simulink model "ASM_Traffic_V2X_Complete_Model_2"  (R2019a)
settings: Solver=ode1  StartTime=SIM.tstart.v  StopTime=Inf  FixedStep=SIM.StepSize.v  RelTol=1e-3
PostLoadFcn:
  | if any(exist('dsrtsu_mdlpostloadfcn', 'file') ~= 0), dsrtsu_mdlpostloadfcn('Execute', bdroot); end
  | try, asm_mdl_postloadfcn(bdroot, 'UpdateModel', 2200); catch, disp(lasterr); end,
undefined symbols (not defined in the file): _SensorPnts_1, _SensorPnts_13, _SensorPnts_17, _SensorPnts_21, _SensorPnts_25, _SensorPnts_29, _SensorPnts_33, _SensorPnts_37, _SensorPnts_41, _SensorPnts_45, _SensorPnts_49, _SensorPnts_5, _SensorPnts_53, _SensorPnts_57, _SensorPnts_9, _to_, CPT, G5A, ITS, MDL, rad, s_to_rpm, SIM
libraries: simulink x169, ASM_VehicleDynamics_lib x126, ASM_Traffic_lib x83, ASM_Utils_lib x49, mdbs x45, ASM_Environment_lib x17, dspindex x12, dsaV2xLibraryAux x10, dsmpblib x6, dsaV2xAsn1Library x4, dsaV2xLibrary x4, ASM_BrakeHydraulics_lib x4
(part 23 of 36)

== system ASM_Traffic_V2X_Complete_Model_2/MDLUserInterface/SoftECU/MDL_DISP/SoftECU_ACC/Dist_Long[m] ==
  In1 : Inport
  Out1 : Outport
  wires:
  In1/1 -> Out1/1

== system ASM_Traffic_V2X_Complete_Model_2/MDLUserInterface/SoftECU/MDL_DISP/SoftECU_ACC/Distance_Set[m] ==
  In1 : Inport
  Out1 : Outport
  wires:
  In1/1 -> Out1/1

== system ASM_Traffic_V2X_Complete_Model_2/MDLUserInterface/SoftECU/MDL_DISP/SoftECU_ACC/FCW[0Off|1On] ==
  In1 : Inport
  Out1 : Outport
  wires:
  In1/1 -> Out1/1

== system ASM_Traffic_V2X_Complete_Model_2/MDLUserInterface/SoftECU/MDL_DISP/SoftECU_ACC/State_ACC[0Off|1On] ==
  In1 : Inport
  Out1 : Outport
  wires:
  In1/1 -> Out1/1

== system ASM_Traffic_V2X_Complete_Model_2/MDLUserInterface/SoftECU/MDL_DISP/SoftECU_ACC/Sw_BrakeMode[1Comfort|2AEBOnly|3AEBOff] ==
  In1 : Inport
  Out1 : Outport
  wires:
  In1/1 -> Out1/1

== system ASM_Traffic_V2X_Complete_Model_2/MDLUserInterface/SoftECU/MDL_DISP/SoftECU_ACC/TTC[s] ==
  In1 : Inport
  Out1 : Outport
  wires:
  In1/1 -> Out1/1

== system ASM_Traffic_V2X_Complete_Model_2/MDLUserInterface/SoftECU/MDL_DISP/SoftECU_ACC/Target_Detected[0|1] ==
  In1 : Inport
  Out1 : Outport
  wires:
  In1/1 -> Out1/1

== system ASM_Traffic_V2X_Complete_Model_2/MDLUserInterface/SoftECU/MDL_DISP/SoftECU_ACC/Trq_Request_Brake_ACC[Nm] ==
  In1 : Inport
  Out1 : Outport
  wires:
  In1/1 -> Out1/1

== system ASM_Traffic_V2X_Complete_Model_2/MDLUserInterface/SoftECU/MDL_DISP/SoftECU_ACC/Trq_Request_Engine_ACC[Nm] ==
  In1 : Inport
  Out1 : Outport
  wires:
  In1/1 -> Out1/1

== system ASM_Traffic_V2X_Complete_Model_2/MDLUserInterface/SoftECU/MDL_DISP/SoftECU_ACC/v_Rel[km|h] ==
  In1 : Inport
  Out1 : Outport
  wires:
  In1/1 -> Out1/1

== system ASM_Traffic_V2X_Complete_Model_2/MDLUserInterface/SoftECU/MDL_DISP/SoftECU_ACC/v_Set[km|h] ==
  In1 : Inport
  Out1 : Outport
  wires:
  In1/1 -> Out1/1

== system ASM_Traffic_V2X_Complete_Model_2/MDLUserInterface/SoftECU/MDL_DISP/SoftECU_Body/Flag_NotPressed_Pedal[0|1] ==
  In1 : Inport
  Out1 : Outport
  wires:
  In1/1 -> Out1/1

== system ASM_Traffic_V2X_Complete_Model_2/MDLUserInterface/SoftECU/MDL_DISP/SoftECU_Body/StartStateButtonLogic ==
  note: State LED is overwritten (set to EngRunning) if start button state is being stimulated and a running engine sttate has been reached
  In1 : Inport
  AND : Logic  AllPortsSameDT=off  OutDataTypeStr=boolean
  Bus Selector : BusSelector  OutputSignals=Sw_Starter_Mode[1Stim|2PermanentOn]
  Bus Selector5 : BusSelector  OutputSignals=State_Engine[0|1|2|3|4]
  EngRunning : simulink/Logic and Bit Operations/Compare To Constant  relop===  const=3.0  OutDataTypeStr=boolean
  StarterPermanantOn : simulink/Logic and Bit Operations/Compare To Constant  relop===  const=2  OutDataTypeStr=boolean
  Switch : Switch  Criteria=u2 ~= 0
  Out1 : Outport
  wires:
  EngRunning/1 -> AND/2
  In1/1 -> Switch/3
  AND/1 -> Switch/2
  StarterPermanantOn/1 -> AND/1
  Switch/1 -> Out1/1
  Bus Selector5/1 -> Switch/1, EngRunning/1  "<State_Engine[0|1|2|3|4]>"
  [TAG_FromIO_Engine] -> Bus Selector5/1
  [TAG_StartButton_Signals] -> Bus Selector/1
  Bus Selector/1 -> StarterPermanantOn/1  "<Sw_Starter_Mode[1Stim|2PermanentOn]>"

== system ASM_Traffic_V2X_Complete_Model_2/MDLUserInterface/SoftECU/MDL_DISP/SoftECU_Body/State_StartButton[-2NotAuthorized|-1PowerOff|0Acc|1PowerOn|2StarterOn|3EngRunning] ==
  In1 : Inport
  Out1 : Outport
  wires:
  In1/1 -> Out1/1

== system ASM_Traffic_V2X_Complete_Model_2/MDLUserInterface/SoftECU/MDL_DISP/SoftECU_Body/Sw_Ignition[0|1] ==
  In1 : Inport
  Out1 : Outport
  wires:
  In1/1 -> Out1/1

== system ASM_Traffic_V2X_Complete_Model_2/MDLUserInterface/SoftECU/MDL_DISP/SoftECU_Body/Sw_StarterReq[0|1] ==
  In1 : Inport
  Out1 : Outport
  wires:
  In1/1 -> Out1/1

== system ASM_Traffic_V2X_Complete_Model_2/MDLUserInterface/SoftECU/MDL_DISP/SoftECU_Brake/Enable_p_Brake_Desired[0|1] ==
  In1 : Inport
  Out1 : Outport
  wires:
  In1/1 -> Out1/1

== system ASM_Traffic_V2X_Complete_Model_2/MDLUserInterface/SoftECU/MDL_DISP/SoftECU_Brake/p_Brake_Desired[bar] ==
  In1 : Inport
  Out1 : Outport
  wires:
  In1/1 -> Out1/1

== system ASM_Traffic_V2X_Complete_Model_2/MDLUserInterface/SoftECU/MDL_DISP/SoftECU_Engine/Enable_TrqDecrease_ESP[0|1] ==
  In1 : Inport
  Out1 : Outport
  wires:
  In1/1 -> Out1/1

== system ASM_Traffic_V2X_Complete_Model_2/MDLUserInterface/SoftECU/MDL_DISP/SoftECU_Engine/Enable_TrqDecrease_Extern[0|1] ==
  In1 : Inport
  Out1 : Outport
  wires:
  In1/1 -> Out1/1

== system ASM_Traffic_V2X_Complete_Model_2/MDLUserInterface/SoftECU/MDL_DISP/SoftECU_Engine/Enable_Trq_Intervention_Fast[0|1] ==
  In1 : Inport
  Out1 : Outport
  wires:
  In1/1 -> Out1/1

== system ASM_Traffic_V2X_Complete_Model_2/MDLUserInterface/SoftECU/MDL_DISP/SoftECU_Engine/Pos_AccPedal[%] ==
  In1 : Inport
  Out1 : Outport
  wires:
  In1/1 -> Out1/1

== system ASM_Traffic_V2X_Complete_Model_2/MDLUserInterface/SoftECU/MDL_DISP/SoftECU_Engine/Pos_AccPedal_Influenced[%] ==
  In1 : Inport
  Out1 : Outport
  wires:
  In1/1 -> Out1/1

== system ASM_Traffic_V2X_Complete_Model_2/MDLUserInterface/SoftECU/MDL_DISP/SoftECU_Engine/Pos_AccPedal_Request_Extern[%] ==
  In1 : Inport
  Out1 : Outport
  wires:
  In1/1 -> Out1/1

== system ASM_Traffic_V2X_Complete_Model_2/MDLUserInterface/SoftECU/MDL_DISP/SoftECU_Engine/Pos_AccPedal_Request_Fast_ESP[%] ==
  In1 : Inport
  Out1 : Outport
  wires:
  In1/1 -> Out1/1

== system ASM_Traffic_V2X_Complete_Model_2/MDLUserInterface/SoftECU/MDL_DISP/SoftECU_Engine/Pos_AccPedal_Request_Slow_ESP[%]1 ==
  In1 : Inport
  Out1 : Outport
  wires:
  In1/1 -> Out1/1

== system ASM_Traffic_V2X_Complete_Model_2/MDLUserInterface/SoftECU/MDL_DISP/SoftECU_Engine/Trq_DecreaseRequest_ESP[Nm] ==
  In1 : Inport
  Out1 : Outport
  wires:
  In1/1 -> Out1/1

== system ASM_Traffic_V2X_Complete_Model_2/MDLUserInterface/SoftECU/MDL_DISP/SoftECU_Engine/Trq_Request_Fast[Nm] ==
  In1 : Inport
  Out1 : Outport
  wires:
  In1/1 -> Out1/1

== system ASM_Traffic_V2X_Complete_Model_2/MDLUserInterface/SoftECU/MDL_DISP/SoftECU_Transmission/Ctrl_Lockup_Clutch[%] ==
  In1 : Inport
  Out1 : Outport
  wires:
  In1/1 -> Out1/1

== system ASM_Traffic_V2X_Complete_Model_2/MDLUserInterface/SoftECU/MDL_DISP/SoftECU_Transmission/Ctrl_Parking_Pawl[0|1] ==
  In1 : Inport
  Out1 : Outport
  wires:
  In1/1 -> Out1/1

== system ASM_Traffic_V2X_Complete_Model_2/MDLUserInterface/SoftECU/MDL_DISP/SoftECU_Transmission/Factor_Trq_Engine_Red[%] ==
  In1 : Inport
  Out1 : Outport
  wires:
  In1/1 -> Out1/1

== system ASM_Traffic_V2X_Complete_Model_2/MDLUserInterface/SoftECU/MDL_DISP/SoftECU_Transmission/Gear[] ==
  In1 : Inport
  Out1 : Outport
  wires:
  In1/1 -> Out1/1

== system ASM_Traffic_V2X_Complete_Model_2/MDLUserInterface/VehicleDynamics/MDL_DISP/Accelerations/a_FL_Wheel[x;y;z][m|s2] ==
  In1 : Inport
  Out1 : Outport
  wires:
  In1/1 -> Out1/1

== system ASM_Traffic_V2X_Complete_Model_2/MDLUserInterface/VehicleDynamics/MDL_DISP/Accelerations/a_FR_Wheel[x;y;z][m|s2] ==
  In1 : Inport
  Out1 : Outport
  wires:
  In1/1 -> Out1/1

== system ASM_Traffic_V2X_Complete_Model_2/MDLUserInterface/VehicleDynamics/MDL_DISP/Accelerations/a_RL_Wheel[x;y;z][m|s2] ==
  In1 : Inport
  Out1 : Outport
  wires:
  In1/1 -> Out1/1

== system ASM_Traffic_V2X_Complete_Model_2/MDLUserInterface/VehicleDynamics/MDL_DISP/Accelerations/a_RR_Wheel[x;y;z][m|s2] ==
  In1 : Inport
  Out1 : Outport
  wires:
  In1/1 -> Out1/1

== system ASM_Traffic_V2X_Complete_Model_2/MDLUserInterface/VehicleDynamics/MDL_DISP/Accelerations/a_x_Vehicle_CoG[m|s2] ==
  In1 : Inport
  Out1 : Outport
  wires:
  In1/1 -> Out1/1

== system ASM_Traffic_V2X_Complete_Model_2/MDLUserInterface/VehicleDynamics/MDL_DISP/Accelerations/a_y_Vehicle_CoG[m|s2] ==
  In1 : Inport
  Out1 : Outport
  wires:
  In1/1 -> Out1/1

== system ASM_Traffic_V2X_Complete_Model_2/MDLUserInterface/VehicleDynamics/MDL_DISP/Accelerations/a_z_Vehicle_CoG[m|s2] ==
  In1 : Inport
  Out1 : Outport
  wires:
  In1/1 -> Out1/1

== system ASM_Traffic_V2X_Complete_Model_2/MDLUserInterface/VehicleDynamics/MDL_DISP/Accelerations/w_Vehicle_CoG_dt[x;y;z][rad|s2] ==
  In1 : Inport
  Out1 : Outport
  wires:
  In1/1 -> Out1/1

== system ASM_Traffic_V2X_Complete_Model_2/MDLUserInterface/VehicleDynamics/MDL_DISP/Accelerations/w_x_Vehicle_CoG_dt[rad|s2] ==
  In1 : Inport
  Out1 : Outport
  wires:
  In1/1 -> Out1/1

== system ASM_Traffic_V2X_Complete_Model_2/MDLUserInterface/VehicleDynamics/MDL_DISP/Accelerations/w_y_Vehicle_CoG_dt[rad|s2] ==
  In1 : Inport
  Out1 : Outport
  wires:
  In1/1 -> Out1/1

== system ASM_Traffic_V2X_Complete_Model_2/MDLUserInterface/VehicleDynamics/MDL_DISP/Accelerations/w_z_Vehicle_CoG_dt[rad|s2] ==
  In1 : Inport
  Out1 : Outport
  wires:
  In1/1 -> Out1/1

== system ASM_Traffic_V2X_Complete_Model_2/MDLUserInterface/VehicleDynamics/MDL_DISP/Aerodynamics/F_x_Aero_CoorSys_V[N] ==
  In1 : Inport
  Out1 : Outport
  wires:
  In1/1 -> Out1/1

== system ASM_Traffic_V2X_Complete_Model_2/MDLUserInterface/VehicleDynamics/MDL_DISP/Aerodynamics/F_y_Aero_CoorSys_V[N] ==
  In1 : Inport
  Out1 : Outport
  wires:
  In1/1 -> Out1/1

== system ASM_Traffic_V2X_Complete_Model_2/MDLUserInterface/VehicleDynamics/MDL_DISP/Aerodynamics/F_z_Aero_CoorSys_V[N] ==
  In1 : Inport
  Out1 : Outport
  wires:
  In1/1 -> Out1/1

== system ASM_Traffic_V2X_Complete_Model_2/MDLUserInterface/VehicleDynamics/MDL_DISP/Aerodynamics/Trq_x_Aero_CoorSys_V[Nm] ==
  In1 : Inport
  Out1 : Outport
  wires:
  In1/1 -> Out1/1

== system ASM_Traffic_V2X_Complete_Model_2/MDLUserInterface/VehicleDynamics/MDL_DISP/Aerodynamics/Trq_y_Aero_CoorSys_V[Nm] ==
  In1 : Inport
  Out1 : Outport
  wires:
  In1/1 -> Out1/1

== system ASM_Traffic_V2X_Complete_Model_2/MDLUserInterface/VehicleDynamics/MDL_DISP/Aerodynamics/Trq_z_Aero_CoorSys_V[Nm] ==
  In1 : Inport
  Out1 : Outport
  wires:
  In1/1 -> Out1/1

== system ASM_Traffic_V2X_Complete_Model_2/MDLUserInterface/VehicleDynamics/MDL_DISP/Brake/BrakeHydraulicsModel[] ==
  In1 : Inport
  Gain : Gain
  Out1 : Outport
  wires:
  In1/1 -> Gain/1
  Gain/1 -> Out1/1

== system ASM_Traffic_V2X_Complete_Model_2/MDLUserInterface/VehicleDynamics/MDL_DISP/Brake/Trq_FL_Brake[Nm] ==
  In1 : Inport
  Out1 : Outport
  wires:
  In1/1 -> Out1/1

== system ASM_Traffic_V2X_Complete_Model_2/MDLUserInterface/VehicleDynamics/MDL_DISP/Brake/Trq_FR_Brake[Nm] ==
  In1 : Inport
  Out1 : Outport
  wires:
  In1/1 -> Out1/1

== system ASM_Traffic_V2X_Complete_Model_2/MDLUserInterface/VehicleDynamics/MDL_DISP/Brake/Trq_RL_Brake[Nm] ==
  In1 : Inport
  Out1 : Outport
  wires:
  In1/1 -> Out1/1

== system ASM_Traffic_V2X_Complete_Model_2/MDLUserInterface/VehicleDynamics/MDL_DISP/Brake/Trq_RR_Brake[Nm] ==
  In1 : Inport
  Out1 : Outport
  wires:
  In1/1 -> Out1/1

== system ASM_Traffic_V2X_Complete_Model_2/MDLUserInterface/VehicleDynamics/MDL_DISP/Brake/p[bar] ==
  In1 : Inport
  Out1 : Outport
  wires:
  In1/1 -> Out1/1

== system ASM_Traffic_V2X_Complete_Model_2/MDLUserInterface/VehicleDynamics/MDL_DISP/Brake/p_FL_Brake[bar] ==
  In1 : Inport
  Out1 : Outport
  wires:
  In1/1 -> Out1/1

== system ASM_Traffic_V2X_Complete_Model_2/MDLUserInterface/VehicleDynamics/MDL_DISP/Brake/p_FR_Brake[bar] ==
  In1 : Inport
  Out1 : Outport
  wires:
  In1/1 -> Out1/1

== system ASM_Traffic_V2X_Complete_Model_2/MDLUserInterface/VehicleDynamics/MDL_DISP/Brake/p_RL_Brake[bar] ==
  In1 : Inport
  Out1 : Outport
  wires:
  In1/1 -> Out1/1

== system ASM_Traffic_V2X_Complete_Model_2/MDLUserInterface/VehicleDynamics/MDL_DISP/Brake/p_RR_Brake[bar] ==
  In1 : Inport
  Out1 : Outport
  wires:
  In1/1 -> Out1/1

== system ASM_Traffic_V2X_Complete_Model_2/MDLUserInterface/VehicleDynamics/MDL_DISP/Brake/p_max[bar] ==
  In1 : Inport
  Out1 : Outport
  wires:
  In1/1 -> Out1/1

== system ASM_Traffic_V2X_Complete_Model_2/MDLUserInterface/VehicleDynamics/MDL_DISP/Overview/a_x_Vehicle_CoG[m|s2] ==
  In1 : Inport
  Out1 : Outport
  wires:
  In1/1 -> Out1/1

== system ASM_Traffic_V2X_Complete_Model_2/MDLUserInterface/VehicleDynamics/MDL_DISP/Overview/a_y_Vehicle_CoG[m|s2] ==
  In1 : Inport
  Out1 : Outport
  wires:
  In1/1 -> Out1/1

== system ASM_Traffic_V2X_Complete_Model_2/MDLUserInterface/VehicleDynamics/MDL_DISP/Overview/a_z_Vehicle_CoG[m|s2] ==
  In1 : Inport
  Out1 : Outport
  wires:
  In1/1 -> Out1/1

== system ASM_Traffic_V2X_Complete_Model_2/MDLUserInterface/VehicleDynamics/MDL_DISP/Overview/v_Total_Vehicle[km|h] ==
  In1 : Inport
  Out1 : Outport
  wires:
  In1/1 -> Out1/1

== system ASM_Traffic_V2X_Complete_Model_2/MDLUserInterface/VehicleDynamics/MDL_DISP/Overview/v_x_Vehicle_CoG[km|h] ==
  In1 : Inport
  Out1 : Outport
  wires:
  In1/1 -> Out1/1

== system ASM_Traffic_V2X_Complete_Model_2/MDLUserInterface/VehicleDynamics/MDL_DISP/Overview/v_y_Vehicle_CoG[km|h] ==
  In1 : Inport
  Out1 : Outport
  wires:
  In1/1 -> Out1/1

== system ASM_Traffic_V2X_Complete_Model_2/MDLUserInterface/VehicleDynamics/MDL_DISP/Overview/v_z_Vehicle_CoG[km|h] ==
  In1 : Inport
  Out1 : Outport
  wires:
  In1/1 -> Out1/1

== system ASM_Traffic_V2X_Complete_Model_2/MDLUserInterface/VehicleDynamics/MDL_DISP/Positions/Angle_Pitch_Vehicle_CoorSys_E[deg] ==
  In1 : Inport
  Out1 : Outport
  wires:
  In1/1 -> Out1/1

== system ASM_Traffic_V2X_Complete_Model_2/MDLUserInterface/VehicleDynamics/MDL_DISP/Positions/Angle_Roll_Vehicle_CoorSys_E[deg] ==
  In1 : Inport
  Out1 : Outport
  wires:
  In1/1 -> Out1/1

== system ASM_Traffic_V2X_Complete_Model_2/MDLUserInterface/VehicleDynamics/MDL_DISP/Positions/Angle_Yaw_Vehicle_CoorSys_E[deg] ==
  In1 : Inport
  Out1 : Outport
  wires:
  In1/1 -> Out1/1

== system ASM_Traffic_V2X_Complete_Model_2/MDLUserInterface/VehicleDynamics/MDL_DISP/Positions/Pos_x_Vehicle_CoorSys_E[m] ==
  In1 : Inport
  Out1 : Outport
  wires:
  In1/1 -> Out1/1

== system ASM_Traffic_V2X_Complete_Model_2/MDLUserInterface/VehicleDynamics/MDL_DISP/Positions/Pos_y_Vehicle_CoorSys_E[m] ==
  In1 : Inport
  Out1 : Outport
  wires:
  In1/1 -> Out1/1

== system ASM_Traffic_V2X_Complete_Model_2/MDLUserInterface/VehicleDynamics/MDL_DISP/Positions/Pos_z_Vehicle_CoorSys_E[m] ==
  In1 : Inport
  Out1 : Outport
  wires:
  In1/1 -> Out1/1

== system ASM_Traffic_V2X_Complete_Model_2/MDLUserInterface/VehicleDynamics/MDL_DISP/Positions/s_Vehicle[m] ==
  In1 : Inport
  Out1 : Outport
  wires:
  In1/1 -> Out1/1

== system ASM_Traffic_V2X_Complete_Model_2/MDLUserInterface/VehicleDynamics/MDL_DISP/Steering/Angle_SteeringGear[deg] ==
  In1 : Inport
  Out1 : Outport
  wires:
  In1/1 -> Out1/1

== system ASM_Traffic_V2X_Complete_Model_2/MDLUserInterface/VehicleDynamics/MDL_DISP/Steering/Angle_SteeringWheel[deg] ==
  In1 : Inport
  Out1 : Outport
  wires:
  In1/1 -> Out1/1

== system ASM_Traffic_V2X_Complete_Model_2/MDLUserInterface/VehicleDynamics/MDL_DISP/Steering/Displ_Steering[m] ==
  In1 : Inport
  Out1 : Outport
  wires:
  In1/1 -> Out1/1

== system ASM_Traffic_V2X_Complete_Model_2/MDLUserInterface/VehicleDynamics/MDL_DISP/Steering/Trq_PowerSteering[Nm] ==
  In1 : Inport
  Out1 : Outport
  wires:
  In1/1 -> Out1/1

== system ASM_Traffic_V2X_Complete_Model_2/MDLUserInterface/VehicleDynamics/MDL_DISP/Steering/Trq_Steering[Nm] ==
  In1 : Inport
  Out1 : Outport
  wires:
  In1/1 -> Out1/1

== system ASM_Traffic_V2X_Complete_Model_2/MDLUserInterface/VehicleDynamics/MDL_DISP/Steering/i_Steering_Mean[] ==
  In1 : Inport
  Out1 : Outport
  wires:
  In1/1 -> Out1/1

== system ASM_Traffic_V2X_Complete_Model_2/MDLUserInterface/VehicleDynamics/MDL_DISP/Suspension/Angle_Alpha_FL_Wheel[deg] ==
  In1 : Inport
  Out1 : Outport
  wires:
  In1/1 -> Out1/1

== system ASM_Traffic_V2X_Complete_Model_2/MDLUserInterface/VehicleDynamics/MDL_DISP/Suspension/Angle_Alpha_FR_Wheel[deg] ==
  In1 : Inport
  Out1 : Outport
  wires:
  In1/1 -> Out1/1

== system ASM_Traffic_V2X_Complete_Model_2/MDLUserInterface/VehicleDynamics/MDL_DISP/Suspension/Angle_Alpha_RL_Wheel[deg] ==
  In1 : Inport
  Out1 : Outport
  wires:
  In1/1 -> Out1/1

== system ASM_Traffic_V2X_Complete_Model_2/MDLUserInterface/VehicleDynamics/MDL_DISP/Suspension/Angle_Alpha_RR_Wheel[deg] ==
  In1 : Inport
  Out1 : Outport
  wires:
  In1/1 -> Out1/1

== system ASM_Traffic_V2X_Complete_Model_2/MDLUserInterface/VehicleDynamics/MDL_DISP/Suspension/Angle_Beta_FL_Wheel[deg] ==
  In1 : Inport
  Out1 : Outport
  wires:
  In1/1 -> Out1/1

== system ASM_Traffic_V2X_Complete_Model_2/MDLUserInterface/VehicleDynamics/MDL_DISP/Suspension/Angle_Beta_FR_Wheel[deg] ==
  In1 : Inport
  Out1 : Outport
  wires:
  In1/1 -> Out1/1

== system ASM_Traffic_V2X_Complete_Model_2/MDLUserInterface/VehicleDynamics/MDL_DISP/Suspension/Angle_Beta_RL_Wheel[deg] ==
  In1 : Inport
  Out1 : Outport
  wires:
  In1/1 -> Out1/1

== system ASM_Traffic_V2X_Complete_Model_2/MDLUserInterface/VehicleDynamics/MDL_DISP/Suspension/Angle_Beta_RR_Wheel[deg] ==
  In1 : Inport
  Out1 : Outport
  wires:
  In1/1 -> Out1/1

== system ASM_Traffic_V2X_Complete_Model_2/MDLUserInterface/VehicleDynamics/MDL_DISP/Suspension/Angle_FL_Wheel[Alpha;Beta;Gamma][deg] ==
  In1 : Inport
  Out1 : Outport
  wires:
  In1/1 -> Out1/1

== system ASM_Traffic_V2X_Complete_Model_2/MDLUserInterface/VehicleDynamics/MDL_DISP/Suspension/Angle_FRWheel[Alpha;Beta;Gamma][deg] ==
  In1 : Inport
  Out1 : Outport
  wires:
  In1/1 -> Out1/1

== system ASM_Traffic_V2X_Complete_Model_2/MDLUserInterface/VehicleDynamics/MDL_DISP/Suspension/Angle_Gamma_FL_Wheel[deg] ==
  In1 : Inport
  Out1 : Outport
  wires:
  In1/1 -> Out1/1

== system ASM_Traffic_V2X_Complete_Model_2/MDLUserInterface/VehicleDynamics/MDL_DISP/Suspension/Angle_Gamma_FR_Wheel[deg] ==
  In1 : Inport
  Out1 : Outport
  wires:
  In1/1 -> Out1/1

== system ASM_Traffic_V2X_Complete_Model_2/MDLUserInterface/VehicleDynamics/MDL_DISP/Suspension/Angle_Gamma_RL_Wheel[deg] ==
  In1 : Inport
  Out1 : Outport
  wires:
  In1/1 -> Out1/1

== system ASM_Traffic_V2X_Complete_Model_2/MDLUserInterface/VehicleDynamics/MDL_DISP/Suspension/Angle_Gamma_RR_Wheel[deg] ==
  In1 : Inport
  Out1 : Outport
  wires:
  In1/1 -> Out1/1

== system ASM_Traffic_V2X_Complete_Model_2/MDLUserInterface/VehicleDynamics/MDL_DISP/Suspension/Angle_RL_Wheel[Alpha;Beta;Gamma][deg] ==
  In1 : Inport
  Out1 : Outport
  wires:
  In1/1 -> Out1/1

== system ASM_Traffic_V2X_Complete_Model_2/MDLUserInterface/VehicleDynamics/MDL_DISP/Suspension/Angle_RR_Wheel[Alpha;Beta;Gamma][deg] ==
  In1 : Inport
  Out1 : Outport
  wires:
  In1/1 -> Out1/1

== system ASM_Traffic_V2X_Complete_Model_2/MDLUserInterface/VehicleDynamics/MDL_DISP/Suspension/Displ_Damper_FL[m] ==
  In1 : Inport
  Out1 : Outport
  wires:
  In1/1 -> Out1/1

== system ASM_Traffic_V2X_Complete_Model_2/MDLUserInterface/VehicleDynamics/MDL_DISP/Suspension/Displ_Damper_FL_dt[m|s] ==
  In1 : Inport
  Out1 : Outport
  wires:
  In1/1 -> Out1/1

== system ASM_Traffic_V2X_Complete_Model_2/MDLUserInterface/VehicleDynamics/MDL_DISP/Suspension/Displ_Damper_FR[m] ==
  In1 : Inport
  Out1 : Outport
  wires:
  In1/1 -> Out1/1

== system ASM_Traffic_V2X_Complete_Model_2/MDLUserInterface/VehicleDynamics/MDL_DISP/Suspension/Displ_Damper_FR_dt[m|s] ==
  In1 : Inport
  Out1 : Outport
  wires:
  In1/1 -> Out1/1

== system ASM_Traffic_V2X_Complete_Model_2/MDLUserInterface/VehicleDynamics/MDL_DISP/Suspension/Displ_Damper_RL[m] ==
  In1 : Inport
  Out1 : Outport
  wires:
  In1/1 -> Out1/1

== system ASM_Traffic_V2X_Complete_Model_2/MDLUserInterface/VehicleDynamics/MDL_DISP/Suspension/Displ_Damper_RL_dt[m|s] ==
  In1 : Inport
  Out1 : Outport
  wires:
  In1/1 -> Out1/1

== system ASM_Traffic_V2X_Complete_Model_2/MDLUserInterface/VehicleDynamics/MDL_DISP/Suspension/Displ_Damper_RR[m] ==
  In1 : Inport
  Out1 : Outport
  wires:
  In1/1 -> Out1/1

== system ASM_Traffic_V2X_Complete_Model_2/MDLUserInterface/VehicleDynamics/MDL_DISP/Suspension/Displ_Damper_RR_dt[m|s] ==
  In1 : Inport
  Out1 : Outport
  wires:
  In1/1 -> Out1/1

== system ASM_Traffic_V2X_Complete_Model_2/MDLUserInterface/VehicleDynamics/MDL_DISP/Suspension/Displ_Spring_FL[m] ==
  In1 : Inport
  Out1 : Outport
  wires:
  In1/1 -> Out1/1

== system ASM_Traffic_V2X_Complete_Model_2/MDLUserInterface/VehicleDynamics/MDL_DISP/Suspension/Displ_Spring_FRm] ==
  In1 : Inport
  Out1 : Outport
  wires:
  In1/1 -> Out1/1

== system ASM_Traffic_V2X_Complete_Model_2/MDLUserInterface/VehicleDynamics/MDL_DISP/Suspension/Displ_Spring_RL[m] ==
  In1 : Inport
  Out1 : Outport
  wires:
  In1/1 -> Out1/1

== system ASM_Traffic_V2X_Complete_Model_2/MDLUserInterface/VehicleDynamics/MDL_DISP/Suspension/Displ_Spring_RR[m] ==
  In1 : Inport
  Out1 : Outport
  wires:
  In1/1 -> Out1/1

== system ASM_Traffic_V2X_Complete_Model_2/MDLUserInterface/VehicleDynamics/MDL_DISP/Suspension/Displ_Stabilizer_Front[m] ==
  In1 : Inport
  Out1 : Outport
  wires:
  In1/1 -> Out1/1

== system ASM_Traffic_V2X_Complete_Model_2/MDLUserInterface/VehicleDynamics/MDL_DISP/Suspension/Displ_Stabilizer_Rear[m] ==
  In1 : Inport
  Out1 : Outport
  wires:
  In1/1 -> Out1/1

== system ASM_Traffic_V2X_Complete_Model_2/MDLUserInterface/VehicleDynamics/MDL_DISP/Suspension/F_FL_Damper[N] ==
  In1 : Inport
  Out1 : Outport
  wires:
  In1/1 -> Out1/1

== system ASM_Traffic_V2X_Complete_Model_2/MDLUserInterface/VehicleDynamics/MDL_DISP/Suspension/F_FL_Spring[N] ==
  In1 : Inport
  Out1 : Outport
  wires:
  In1/1 -> Out1/1

== system ASM_Traffic_V2X_Complete_Model_2/MDLUserInterface/VehicleDynamics/MDL_DISP/Suspension/F_FR_Damper[N] ==
  In1 : Inport
  Out1 : Outport
  wires:
  In1/1 -> Out1/1

== system ASM_Traffic_V2X_Complete_Model_2/MDLUserInterface/VehicleDynamics/MDL_DISP/Suspension/F_FR_Spring[N] ==
  In1 : Inport
  Out1 : Outport
  wires:
  In1/1 -> Out1/1

== system ASM_Traffic_V2X_Complete_Model_2/MDLUserInterface/VehicleDynamics/MDL_DISP/Suspension/F_RL_Damper[N] ==
  In1 : Inport
  Out1 : Outport
  wires:
  In1/1 -> Out1/1

== system ASM_Traffic_V2X_Complete_Model_2/MDLUserInterface/VehicleDynamics/MDL_DISP/Suspension/F_RL_Spring[N] ==
  In1 : Inport
  Out1 : Outport
  wires:
  In1/1 -> Out1/1

== system ASM_Traffic_V2X_Complete_Model_2/MDLUserInterface/VehicleDynamics/MDL_DISP/Suspension/F_RR_Damper[N] ==
  In1 : Inport
  Out1 : Outport
  wires:
  In1/1 -> Out1/1

== system ASM_Traffic_V2X_Complete_Model_2/MDLUserInterface/VehicleDynamics/MDL_DISP/Suspension/F_RR_Spring[N] ==
  In1 : Inport
  Out1 : Outport
  wires:
  In1/1 -> Out1/1

== system ASM_Traffic_V2X_Complete_Model_2/MDLUserInterface/VehicleDynamics/MDL_DISP/Suspension/F_Stabilizer_Front[N] ==
  In1 : Inport
  Out1 : Outport
  wires:
  In1/1 -> Out1/1

== system ASM_Traffic_V2X_Complete_Model_2/MDLUserInterface/VehicleDynamics/MDL_DISP/Suspension/F_Stabilizer_Rear[N] ==
  In1 : Inport
  Out1 : Outport
  wires:
  In1/1 -> Out1/1

== system ASM_Traffic_V2X_Complete_Model_2/MDLUserInterface/VehicleDynamics/MDL_DISP/Suspension/Pos_FL_Wheel[x;y;z][m] ==
  In1 : Inport
  Out1 : Outport
  wires:
  In1/1 -> Out1/1

== system ASM_Traffic_V2X_Complete_Model_2/MDLUserInterface/VehicleDynamics/MDL_DISP/Suspension/Pos_FR_Wheel[x;y;z][m] ==
  In1 : Inport
  Out1 : Outport
  wires:
  In1/1 -> Out1/1

== system ASM_Traffic_V2X_Complete_Model_2/MDLUserInterface/VehicleDynamics/MDL_DISP/Suspension/Pos_RL_Wheel[x;y;z][m] ==
  In1 : Inport
  Out1 : Outport
  wires:
  In1/1 -> Out1/1

== system ASM_Traffic_V2X_Complete_Model_2/MDLUserInterface/VehicleDynamics/MDL_DISP/Suspension/Pos_RR_Wheel[x;y;z][m] ==
  In1 : Inport
  Out1 : Outport
  wires:
  In1/1 -> Out1/1

== system ASM_Traffic_V2X_Complete_Model_2/MDLUserInterface/VehicleDynamics/MDL_DISP/Suspension/SusKinFrontModel[] ==
  In1 : Inport
  Gain : Gain
  Out1 : Outport
  wires:
  Gain/1 -> Out1/1
  In1/1 -> Gain/1

== system ASM_Traffic_V2X_Complete_Model_2/MDLUserInterface/VehicleDynamics/MDL_DISP/Suspension/SusKinRearModel[] ==
  In1 : Inport
  Gain : Gain
  Out1 : Outport
  wires:
  Gain/1 -> Out1/1
  In1/1 -> Gain/1

== system ASM_Traffic_V2X_Complete_Model_2/MDLUserInterface/VehicleDynamics/MDL_DISP/Tire/F_x_Dyn_FL_Tire_CoorSys_CP[N] ==
  In1 : Inport
  Out1 : Outport
  wires:
  In1/1 -> Out1/1

== system ASM_Traffic_V2X_Complete_Model_2/MDLUserInterface/VehicleDynamics/MDL_DISP/Tire/F_x_Dyn_FR_Tire_CoorSys_CP[N] ==
  In1 : Inport
  Out1 : Outport
  wires:
  In1/1 -> Out1/1

== system ASM_Traffic_V2X_Complete_Model_2/MDLUserInterface/VehicleDynamics/MDL_DISP/Tire/F_x_Dyn_RL_Tire_CoorSys_CP[N] ==
  In1 : Inport
  Out1 : Outport
  wires:
  In1/1 -> Out1/1

== system ASM_Traffic_V2X_Complete_Model_2/MDLUserInterface/VehicleDynamics/MDL_DISP/Tire/F_x_Dyn_RR_Tire_CoorSys_CP[N] ==
  In1 : Inport
  Out1 : Outport
  wires:
  In1/1 -> Out1/1

== system ASM_Traffic_V2X_Complete_Model_2/MDLUserInterface/VehicleDynamics/MDL_DISP/Tire/F_y_Dyn_FL_Tire_CoorSys_CP[N] ==
  In1 : Inport
  Out1 : Outport
  wires:
  In1/1 -> Out1/1

== system ASM_Traffic_V2X_Complete_Model_2/MDLUserInterface/VehicleDynamics/MDL_DISP/Tire/F_y_Dyn_FR_Tire_CoorSys_CP[N] ==
  In1 : Inport
  Out1 : Outport
  wires:
  In1/1 -> Out1/1

== system ASM_Traffic_V2X_Complete_Model_2/MDLUserInterface/VehicleDynamics/MDL_DISP/Tire/F_y_Dyn_RL_Tire_CoorSys_CP[N] ==
  In1 : Inport
  Out1 : Outport
  wires:
  In1/1 -> Out1/1

== system ASM_Traffic_V2X_Complete_Model_2/MDLUserInterface/VehicleDynamics/MDL_DISP/Tire/F_y_Dyn_RR_Tire_CoorSys_CP[N] ==
  In1 : Inport
  Out1 : Outport
  wires:
  In1/1 -> Out1/1

== system ASM_Traffic_V2X_Complete_Model_2/MDLUserInterface/VehicleDynamics/MDL_DISP/Tire/F_z_Dyn_FL_Tire_CoorSys_CP[N] ==
  In1 : Inport
  Out1 : Outport
  wires:
  In1/1 -> Out1/1

== system ASM_Traffic_V2X_Complete_Model_2/MDLUserInterface/VehicleDynamics/MDL_DISP/Tire/F_z_Dyn_FR_Tire_CoorSys_CP[N] ==
  In1 : Inport
  Out1 : Outport
  wires:
  In1/1 -> Out1/1

== system ASM_Traffic_V2X_Complete_Model_2/MDLUserInterface/VehicleDynamics/MDL_DISP/Tire/F_z_Dyn_RL_Tire_CoorSys_CP[N] ==
  In1 : Inport
  Out1 : Outport
  wires:
  In1/1 -> Out1/1

== system ASM_Traffic_V2X_Complete_Model_2/MDLUserInterface/VehicleDynamics/MDL_DISP/Tire/F_z_Dyn_RR_Tire_CoorSys_CP[N] ==
  In1 : Inport
  Out1 : Outport
  wires:
  In1/1 -> Out1/1

== system ASM_Traffic_V2X_Complete_Model_2/MDLUserInterface/VehicleDynamics/MDL_DISP/Tire/Slip_x_FL[] ==
  In1 : Inport
  Out1 : Outport
  wires:
  In1/1 -> Out1/1

== system ASM_Traffic_V2X_Complete_Model_2/MDLUserInterface/VehicleDynamics/MDL_DISP/Tire/Slip_x_FR[] ==
  In1 : Inport
  Out1 : Outport
  wires:
  In1/1 -> Out1/1

== system ASM_Traffic_V2X_Complete_Model_2/MDLUserInterface/VehicleDynamics/MDL_DISP/Tire/Slip_x_RL[] ==
  In1 : Inport
  Out1 : Outport
  wires:
  In1/1 -> Out1/1

== system ASM_Traffic_V2X_Complete_Model_2/MDLUserInterface/VehicleDynamics/MDL_DISP/Tire/Slip_x_RR[] ==
  In1 : Inport
  Out1 : Outport
  wires:
  In1/1 -> Out1/1

== system ASM_Traffic_V2X_Complete_Model_2/MDLUserInterface/VehicleDynamics/MDL_DISP/Tire/Slip_y_FL[] ==
  In1 : Inport
  Out1 : Outport
  wires:
  In1/1 -> Out1/1

== system ASM_Traffic_V2X_Complete_Model_2/MDLUserInterface/VehicleDynamics/MDL_DISP/Tire/Slip_y_FR[] ==
  In1 : Inport
  Out1 : Outport
  wires:
  In1/1 -> Out1/1

== system ASM_Traffic_V2X_Complete_Model_2/MDLUserInterface/VehicleDynamics/MDL_DISP/Tire/Slip_y_RL[] ==
  In1 : Inport
  Out1 : Outport
  wires:
  In1/1 -> Out1/1

== system ASM_Traffic_V2X_Complete_Model_2/MDLUserInterface/VehicleDynamics/MDL_DISP/Tire/Slip_y_RR[] ==
  In1 : Inport
  Out1 : Outport
  wires:
  In1/1 -> Out1/1

== system ASM_Traffic_V2X_Complete_Model_2/MDLUserInterface/VehicleDynamics/MDL_DISP/Tire/Trq_x_FL_CoorSys_CP[Nm] ==
  In1 : Inport
  Out1 : Outport
  wires:
  In1/1 -> Out1/1

== system ASM_Traffic_V2X_Complete_Model_2/MDLUserInterface/VehicleDynamics/MDL_DISP/Tire/Trq_x_FR_CoorSys_CP[Nm] ==
  In1 : Inport
  Out1 : Outport
  wires:
  In1/1 -> Out1/1

== system ASM_Traffic_V2X_Complete_Model_2/MDLUserInterface/VehicleDynamics/MDL_DISP/Tire/Trq_x_RL_CoorSys_CP[Nm] ==
  In1 : Inport
  Out1 : Outport
  wires:
  In1/1 -> Out1/1

== system ASM_Traffic_V2X_Complete_Model_2/MDLUserInterface/VehicleDynamics/MDL_DISP/Tire/Trq_x_RR_CoorSys_CP[Nm] ==
  In1 : Inport
  Out1 : Outport
  wires:
  In1/1 -> Out1/1

== system ASM_Traffic_V2X_Complete_Model_2/MDLUserInterface/VehicleDynamics/MDL_DISP/Tire/Trq_y_FL_CoorSys_W[Nm] ==
  In1 : Inport
  Out1 : Outport
  wires:
  In1/1 -> Out1/1

== system ASM_Traffic_V2X_Complete_Model_2/MDLUserInterface/VehicleDynamics/MDL_DISP/Tire/Trq_y_FR_CoorSys_W[Nm] ==
  In1 : Inport
  Out1 : Outport
  wires:
  In1/1 -> Out1/1

== system ASM_Traffic_V2X_Complete_Model_2/MDLUserInterface/VehicleDynamics/MDL_DISP/Tire/Trq_y_RL_CoorSys_W[Nm] ==
  In1 : Inport
  Out1 : Outport
  wires:
  In1/1 -> Out1/1

== system ASM_Traffic_V2X_Complete_Model_2/MDLUserInterface/VehicleDynamics/MDL_DISP/Tire/Trq_y_RR_CoorSys_W[Nm] ==
  In1 : Inport
  Out1 : Outport
  wires:
  In1/1 -> Out1/1

== system ASM_Traffic_V2X_Complete_Model_2/MDLUserInterface/VehicleDynamics/MDL_DISP/Tire/Trq_z_FL_CoorSys_CP[Nm] ==
  In1 : Inport
  Out1 : Outport
  wires:
  In1/1 -> Out1/1

== system ASM_Traffic_V2X_Complete_Model_2/MDLUserInterface/VehicleDynamics/MDL_DISP/Tire/Trq_z_FR_CoorSys_CP[Nm] ==
  In1 : Inport
  Out1 : Outport
  wires:
  In1/1 -> Out1/1

== system ASM_Traffic_V2X_Complete_Model_2/MDLUserInterface/VehicleDynamics/MDL_DISP/Tire/Trq_z_RL_CoorSys_CP[Nm] ==
  In1 : Inport
  Out1 : Outport
  wires:
  In1/1 -> Out1/1

== system ASM_Traffic_V2X_Complete_Model_2/MDLUserInterface/VehicleDynamics/MDL_DISP/Tire/Trq_z_RR_CoorSys_CP[Nm] ==
  In1 : Inport
  Out1 : Outport
  wires:
  In1/1 -> Out1/1

== system ASM_Traffic_V2X_Complete_Model_2/MDLUserInterface/VehicleDynamics/MDL_DISP/Tire/r_Dyn_FL_Tire[m] ==
  In1 : Inport
  Out1 : Outport
  wires:
  In1/1 -> Out1/1

== system ASM_Traffic_V2X_Complete_Model_2/MDLUserInterface/VehicleDynamics/MDL_DISP/Tire/r_Dyn_FR_Tire[m] ==
  In1 : Inport
  Out1 : Outport
  wires:
  In1/1 -> Out1/1

== system ASM_Traffic_V2X_Complete_Model_2/MDLUserInterface/VehicleDynamics/MDL_DISP/Tire/r_Dyn_RL_Tire[m] ==
  In1 : Inport
  Out1 : Outport
  wires:
  In1/1 -> Out1/1

== system ASM_Traffic_V2X_Complete_Model_2/MDLUserInterface/VehicleDynamics/MDL_DISP/Tire/r_Dyn_RR_Tire[m] ==
  In1 : Inport
  Out1 : Outport
  wires:
  In1/1 -> Out1/1

== system ASM_Traffic_V2X_Complete_Model_2/MDLUserInterface/VehicleDynamics/MDL_DISP/Tire/v_Circumf_Dyn_FL_Wheel[km|h] ==
  In1 : Inport
  Out1 : Outport
  wires:
  In1/1 -> Out1/1

== system ASM_Traffic_V2X_Complete_Model_2/MDLUserInterface/VehicleDynamics/MDL_DISP/Tire/v_Circumf_Dyn_FR_Wheel[km|h] ==
  In1 : Inport
  Out1 : Outport
  wires:
  In1/1 -> Out1/1

== system ASM_Traffic_V2X_Complete_Model_2/MDLUserInterface/VehicleDynamics/MDL_DISP/Tire/v_Circumf_Dyn_RL_Wheel[km|h] ==
  In1 : Inport
  Out1 : Outport
  wires:
  In1/1 -> Out1/1

== system ASM_Traffic_V2X_Complete_Model_2/MDLUserInterface/VehicleDynamics/MDL_DISP/Tire/v_Circumf_Dyn_RR_Wheel[km|h] ==
  In1 : Inport
  Out1 : Outport
  wires:
  In1/1 -> Out1/1

== system ASM_Traffic_V2X_Complete_Model_2/MDLUserInterface/VehicleDynamics/MDL_DISP/Velocities/Angle_SideSlip_Vehicle[deg] ==
  In1 : Inport
  Out1 : Outport
  wires:
  In1/1 -> Out1/1

== system ASM_Traffic_V2X_Complete_Model_2/MDLUserInterface/VehicleDynamics/MDL_DISP/Velocities/PitchRate_Vehicle_CoG[deg|s] ==
  In1 : Inport
  Out1 : Outport
  wires:
  In1/1 -> Out1/1

== system ASM_Traffic_V2X_Complete_Model_2/MDLUserInterface/VehicleDynamics/MDL_DISP/Velocities/RollRate_Vehicle_CoG[deg|s] ==
  In1 : Inport
  Out1 : Outport
  wires:
  In1/1 -> Out1/1

== system ASM_Traffic_V2X_Complete_Model_2/MDLUserInterface/VehicleDynamics/MDL_DISP/Velocities/YawRate_Vehicle_CoG[deg|s] ==
  In1 : Inport
  Out1 : Outport
  wires:
  In1/1 -> Out1/1

== system ASM_Traffic_V2X_Complete_Model_2/MDLUserInterface/VehicleDynamics/MDL_DISP/Velocities/v_x_Vehicle_CoG[km|h] ==
  In1 : Inport
  Out1 : Outport
  wires:
  In1/1 -> Out1/1

== system ASM_Traffic_V2X_Complete_Model_2/MDLUserInterface/VehicleDynamics/MDL_DISP/Velocities/v_y_Vehicle_CoG[km|h] ==
  In1 : Inport
  Out1 : Outport
  wires:
  In1/1 -> Out1/1

== system ASM_Traffic_V2X_Complete_Model_2/MDLUserInterface/VehicleDynamics/MDL_DISP/Velocities/v_z_Vehicle_CoG[km|h] ==
  In1 : Inport
  Out1 : Outport
  wires:
  In1/1 -> Out1/1

== system ASM_Traffic_V2X_Complete_Model_2/MDLUserInterface/VehicleDynamics/MDL_DISP/WheelSpeeds/omega_FL_Wheel[rad|s] ==
  In1 : Inport
  Out1 : Outport
  wires:
  In1/1 -> Out1/1

== system ASM_Traffic_V2X_Complete_Model_2/MDLUserInterface/VehicleDynamics/MDL_DISP/WheelSpeeds/omega_FR_Wheel[rad|s] ==
  In1 : Inport
  Out1 : Outport
  wires:
  In1/1 -> Out1/1

== system ASM_Traffic_V2X_Complete_Model_2/MDLUserInterface/VehicleDynamics/MDL_DISP/WheelSpeeds/omega_RL_Wheel[rad|s] ==
  In1 : Inport
  Out1 : Outport
  wires:
  In1/1 -> Out1/1

== system ASM_Traffic_V2X_Complete_Model_2/MDLUserInterface/VehicleDynamics/MDL_DISP/WheelSpeeds/omega_RR_Wheel[rad|s] ==
  In1 : Inport
  Out1 : Outport
  wires:
  In1/1 -> Out1/1

== system ASM_Traffic_V2X_Complete_Model_2/IO/I//O_Subsystem/Bus Configuration (1) - In/Simulated ECUs/DrivekitCAN/Drivekit ==
  Input : Inport
  TX : Subsystem
  _Drivekit_ : BusCreator  Inputs=1
  Drivekit : Outport
  wires:
  _Drivekit_/1 -> Drivekit/1  "Drivekit"
  TX/1(TX) -> _Drivekit_/1  "TX"
  Input/1 -> TX/1(Input)

== system ASM_Traffic_V2X_Complete_Model_2/IO/I//O_Subsystem/Bus Configuration (1) - Out/Simulated ECUs/DrivekitCAN/Drivekit ==
  Drivekit : Inport
  RX : Subsystem
  _Drivekit_ : BusSelector  OutputSignals=RX
  wires:
  Drivekit/1 -> _Drivekit_/1  "Drivekit"
  _Drivekit_/1 -> RX/1(RX)  "<RX>"

== system ASM_Traffic_V2X_Complete_Model_2/IO/V2X_Subsystem/CAM-DENM_Message_Generation/DENM/Create_DENM/dsaV2xBusAdapter_a_BL2 ==
  Status : Inport
  Length : Inport  Port=2
  Data : Inport  Port=3
  Bus Creator : BusCreator  Inputs=3
  Data Type Conversion : DataTypeConversion
  Data Type Conversion1 : DataTypeConversion
  V2X-Bus : Outport
  wires:
  Data Type Conversion1/1 -> Bus Creator/1  "Status"
  Data Type Conversion/1 -> Bus Creator/2  "Length"
  Data/1 -> Bus Creator/3  "Data"
  Status/1 -> Data Type Conversion1/1
  Length/1 -> Data Type Conversion/1
  Bus Creator/1 -> V2X-Bus/1

== system ASM_Traffic_V2X_Complete_Model_2/IO/V2X_Subsystem/CAM-DENM_Message_Generation/Fellow_CAM_1/Create_CAM/PathHistory_PathPoints ==
  Latitude [deg] : Inport
  Longitude [deg] : Inport  Port=2
  Time [s] : Inport  Port=3
  Trigger : TriggerPort  VariantControl=(inherit)  PortDimensions=1
  Constant : Constant
  Delay{3,5,8..9,15,18,25..26,31,38,41,44} (12 alike) : Delay  DelayLength=1  InitialCondition=0
  Sum{,1..2,10..12,20..22} (9 alike) : Sum  Inputs=-+
  posGain_BL2 : Gain  Gain=10
  posGain_BL3 : Gain  Gain=100
  posGain_BL4 : Gain  Gain=10
  if_PathPoint1 : Outport
  deltaLatitude1 : Outport  Port=2
  deltaLongitude1 : Outport  Port=3
  pathDeltaTime1 : Outport  Port=4
  if_PathPoint2 : Outport  Port=5
  deltaLatitude2 : Outport  Port=6
  deltaLongitude2 : Outport  Port=7
  pathDeltaTime2 : Outport  Port=8
  if_PathPoint3 : Outport  Port=9
  deltaLatitude3 : Outport  Port=10
  deltaLongitude3 : Outport  Port=11
  pathDeltaTime3 : Outport  Port=12
  wires:
  Constant/1 -> Delay44/1
  Delay41/1 -> if_PathPoint3/1
  Delay38/1 -> Delay41/1, if_PathPoint2/1
  Delay44/1 -> Delay38/1, if_PathPoint1/1
  posGain_BL2/1 -> Sum20/2, Sum21/2, Sum22/2, Delay31/1
  Delay26/1 -> Sum22/1
  Sum22/1 -> deltaLatitude3/1
  Delay25/1 -> Sum21/1, Delay26/1
  Sum21/1 -> deltaLatitude2/1
  Sum20/1 -> deltaLatitude1/1
  Delay31/1 -> Sum20/1, Delay25/1
  Latitude [deg]/1 -> posGain_BL2/1
  posGain_BL4/1 -> Delay8/1, Sum12/2, Sum11/2, Sum10/2
  Delay5/1 -> Sum12/1
  Sum12/1 -> deltaLongitude3/1
  Delay18/1 -> Delay5/1, Sum11/1
  Sum11/1 -> deltaLongitude2/1
  Sum10/1 -> deltaLongitude1/1
  Delay8/1 -> Delay18/1, Sum10/1
  Longitude [deg]/1 -> posGain_BL4/1
  posGain_BL3/1 -> Sum/2, Sum1/2, Sum2/2, Delay3/1
  Delay15/1 -> Sum2/1
  Sum2/1 -> pathDeltaTime3/1
  Delay9/1 -> Sum1/1, Delay15/1
  Sum1/1 -> pathDeltaTime2/1
  Sum/1 -> pathDeltaTime1/1
  Delay3/1 -> Sum/1, Delay9/1
  Time [s]/1 -> posGain_BL3/1

== system ASM_Traffic_V2X_Complete_Model_2/IO/V2X_Subsystem/CAM-DENM_Message_Generation/Fellow_CAM_2/Create_CAM/PathHistory_PathPoints ==
  Latitude [deg] : Inport
  Longitude [deg] : Inport  Port=2
  Time [s] : Inport  Port=3
  Trigger : TriggerPort  VariantControl=(inherit)  PortDimensions=1
  Constant : Constant
  Delay{3,5,8..9,15,18,25..26,31,38,41,44} (12 alike) : Delay  DelayLength=1  InitialCondition=0
  Sum{,1..2,10..12,20..22} (9 alike) : Sum  Inputs=-+
  posGain_BL2 : Gain  Gain=10
  posGain_BL3 : Gain  Gain=100
  posGain_BL4 : Gain  Gain=10
  if_PathPoint1 : Outport
  deltaLatitude1 : Outport  Port=2
  deltaLongitude1 : Outport  Port=3
  pathDeltaTime1 : Outport  Port=4
  if_PathPoint2 : Outport  Port=5
  deltaLatitude2 : Outport  Port=6
  deltaLongitude2 : Outport  Port=7
  pathDeltaTime2 : Outport  Port=8
  if_PathPoint3 : Outport  Port=9
  deltaLatitude3 : Outport  Port=10
  deltaLongitude3 : Outport  Port=11
  pathDeltaTime3 : Outport  Port=12
  wires:
  Constant/1 -> Delay44/1
  Delay41/1 -> if_PathPoint3/1
  Delay38/1 -> Delay41/1, if_PathPoint2/1
  Delay44/1 -> Delay38/1, if_PathPoint1/1
  posGain_BL2/1 -> Sum20/2, Sum21/2, Sum22/2, Delay31/1
  Delay26/1 -> Sum22/1
  Sum22/1 -> deltaLatitude3/1
  Delay25/1 -> Sum21/1, Delay26/1
  Sum21/1 -> deltaLatitude2/1
  Sum20/1 -> deltaLatitude1/1
  Delay31/1 -> Sum20/1, Delay25/1
  Latitude [deg]/1 -> posGain_BL2/1
  posGain_BL4/1 -> Delay8/1, Sum12/2, Sum11/2, Sum10/2
  Delay5/1 -> Sum12/1
  Sum12/1 -> deltaLongitude3/1
  Delay18/1 -> Delay5/1, Sum11/1
  Sum11/1 -> deltaLongitude2/1
  Sum10/1 -> deltaLongitude1/1
  Delay8/1 -> Delay18/1, Sum10/1
  Longitude [deg]/1 -> posGain_BL4/1
  posGain_BL3/1 -> Sum/2, Sum1/2, Sum2/2, Delay3/1
  Delay15/1 -> Sum2/1
  Sum2/1 -> pathDeltaTime3/1
  Delay9/1 -> Sum1/1, Delay15/1
  Sum1/1 -> pathDeltaTime2/1
  Sum/1 -> pathDeltaTime1/1
  Delay3/1 -> Sum/1, Delay9/1
  Time [s]/1 -> posGain_BL3/1

== system ASM_Traffic_V2X_Complete_Model_2/IO/V2X_Subsystem/CAM-DENM_Message_Generation/Fellow_CAM_3/Create_CAM/PathHistory_PathPoints ==
  Latitude [deg] : Inport
  Longitude [deg] : Inport  Port=2
  Time [s] : Inport  Port=3
  Trigger : TriggerPort  VariantControl=(inherit)  PortDimensions=1
  Constant : Constant
  Delay{3,5,8..9,15,18,25..26,31,38,41,44} (12 alike) : Delay  DelayLength=1  InitialCondition=0
  Sum{,1..2,10..12,20..22} (9 alike) : Sum  Inputs=-+
  posGain_BL2 : Gain  Gain=10
  posGain_BL3 : Gain  Gain=100
  posGain_BL4 : Gain  Gain=10
  if_PathPoint1 : Outport
  deltaLatitude1 : Outport  Port=2
  deltaLongitude1 : Outport  Port=3
  pathDeltaTime1 : Outport  Port=4
  if_PathPoint2 : Outport  Port=5
  deltaLatitude2 : Outport  Port=6
  deltaLongitude2 : Outport  Port=7
  pathDeltaTime2 : Outport  Port=8
  if_PathPoint3 : Outport  Port=9
  deltaLatitude3 : Outport  Port=10
  deltaLongitude3 : Outport  Port=11
  pathDeltaTime3 : Outport  Port=12
  wires:
  Constant/1 -> Delay44/1
  Delay41/1 -> if_PathPoint3/1
  Delay38/1 -> Delay41/1, if_PathPoint2/1
  Delay44/1 -> Delay38/1, if_PathPoint1/1
  posGain_BL2/1 -> Sum20/2, Sum21/2, Sum22/2, Delay31/1
  Delay26/1 -> Sum22/1
  Sum22/1 -> deltaLatitude3/1
  Delay25/1 -> Sum21/1, Delay26/1
  Sum21/1 -> deltaLatitude2/1
  Sum20/1 -> deltaLatitude1/1
  Delay31/1 -> Sum20/1, Delay25/1
  Latitude [deg]/1 -> posGain_BL2/1
  posGain_BL4/1 -> Delay8/1, Sum12/2, Sum11/2, Sum10/2
  Delay5/1 -> Sum12/1
  Sum12/1 -> deltaLongitude3/1
  Delay18/1 -> Delay5/1, Sum11/1
  Sum11/1 -> deltaLongitude2/1
  Sum10/1 -> deltaLongitude1/1
  Delay8/1 -> Delay18/1, Sum10/1
  Longitude [deg]/1 -> posGain_BL4/1
  posGain_BL3/1 -> Sum/2, Sum1/2, Sum2/2, Delay3/1
  Delay15/1 -> Sum2/1
  Sum2/1 -> pathDeltaTime3/1
  Delay9/1 -> Sum1/1, Delay15/1
  Sum1/1 -> pathDeltaTime2/1
  Sum/1 -> pathDeltaTime1/1
  Delay3/1 -> Sum/1, Delay9/1
  Time [s]/1 -> posGain_BL3/1

== system ASM_Traffic_V2X_Complete_Model_2/MDL/Drivetrain/Final_Drive_Assembly/ASMSignalCollector/Clutch_4WD/Dummy_Clutch_4WD ==
  BusCreator : BusCreator  Inputs=3
  Dummy_Trq_Lock_Clutch_4WD : Constant  Value=0
  Dummy_omega_Clutch_4WD_In : Constant  Value=0
  Dummy_omega_Clutch_4WD_Out : Constant  Value=0
  Out : Outport
  wires:
  Dummy_omega_Clutch_4WD_In/1 -> BusCreator/2  "omega_Clutch_4WD_In[rad|s]"
  Dummy_omega_Clutch_4WD_Out/1 -> BusCreator/3  "omega_Clutch_4WD_Out[rad|s]"
  BusCreator/1 -> Out/1  "Clutch_4WD"
  Dummy_Trq_Lock_Clutch_4WD/1 -> BusCreator/1  "Trq_Lock_Clutch_4WD[Nm]"

== system ASM_Traffic_V2X_Complete_Model_2/MDL/Drivetrain/Final_Drive_Assembly/ASMSignalCollector/FinalDrive_Ratio/FinalDriveRatio ==
  Sw_DrivetrainMode[1|2|3] : Inport
  CentralDifferential : Inport  Port=2
  RearDifferential : Inport  Port=3
  FrontDifferential : Inport  Port=4
  Bus Selector : BusSelector  OutputSignals=Const_i_MainReductionGear[],Const_TrqDistribution[]
  Bus Selector1 : BusSelector  OutputSignals=Const_i_MainReductionGear[]
  Bus Selector2 : BusSelector  OutputSignals=Const_i_MainReductionGear[]
  Fcn : Fcn  Expr=1-u[1]
  Product1 : Product  Inputs=**  SaturateOnIntegerOverflow=on  OutDataTypeStr=Inherit: Same as first input
  Product2 : Product  Inputs=**  SaturateOnIntegerOverflow=on  OutDataTypeStr=Inherit: Same as first input
  Product3 : Product  Inputs=**  SaturateOnIntegerOverflow=on  OutDataTypeStr=Inherit: Same as first input
  Sum : Sum  Inputs=|++  SaturateOnIntegerOverflow=on
  Switch : MultiPortSwitch  SaturateOnIntegerOverflow=on
  i_FinalDrive[] : Outport
  wires:
  Switch/1 -> i_FinalDrive[]/1  "i_FinalDrive[]"
  RearDifferential/1 -> Bus Selector2/1
  FrontDifferential/1 -> Bus Selector1/1
  CentralDifferential/1 -> Bus Selector/1
  Product3/1 -> Switch/2
  Sw_DrivetrainMode[1|2|3]/1 -> Switch/1
  Sum/1 -> Product3/2
  Bus Selector/1 -> Product3/1  "<Const_i_MainReductionGear[]>"
  Product2/1 -> Sum/2
  Product1/1 -> Sum/1
  Bus Selector2/1 -> Switch/4, Product2/2  "<Const_i_MainReductionGear[]>"
  Fcn/1 -> Product2/1
  Bus Selector/2 -> Product1/1, Fcn/1  "<Const_TrqDistribution[]>"
  Bus Selector1/1 -> Product1/2, Switch/3  "<Const_i_MainReductionGear[]>"

== system ASM_Traffic_V2X_Complete_Model_2/MDL/Drivetrain/Final_Drive_Assembly/ASMSignalCollector/FinalDrive_Ratio/FinalDriveRatio_FF_FF4WD ==
  FrontDifferential : Inport
  Bus Selector1 : BusSelector  OutputSignals=Const_i_MainReductionGear[]
  FinalDriveRatio[]_ : Subsystem
  i_FinalDrive[] : Outport
  wires:
  FrontDifferential/1 -> Bus Selector1/1
  FinalDriveRatio[]_/1(Out) -> i_FinalDrive[]/1  "i_FinalDrive[]"
  Bus Selector1/1 -> FinalDriveRatio[]_/1(In1)  "<Const_i_MainReductionGear[]>"

== system ASM_Traffic_V2X_Complete_Model_2/MDL/Drivetrain/Final_Drive_Assembly/ASMSignalCollector/Shaft_CF/Dummy_CF_Shaft ==
  BusCreator1 : BusCreator  Inputs=2
  Dummy_Trq_CR_Shaft : Constant  Value=0
  Dummy_omega_Delta_CF_Shaft : Constant  Value=0
  Out : Outport
  wires:
  BusCreator1/1 -> Out/1  "Shaft_CF"
  Dummy_Trq_CR_Shaft/1 -> BusCreator1/1  "Trq_CF_Shaft[Nm]"
  Dummy_omega_Delta_CF_Shaft/1 -> BusCreator1/2  "omega_Delta_CF_Shaft[rad|s]"

== system ASM_Traffic_V2X_Complete_Model_2/MDL/Drivetrain/Final_Drive_Assembly/ASMSignalCollector/Shaft_CR/Dummy_CR_Shaft ==
  BusCreator1 : BusCreator  Inputs=2
  Dummy_Trq_CR_Shaft : Constant  Value=0
  Dummy_omega_Delta_CR_Shaft : Constant  Value=0
  Out : Outport
  wires:
  Dummy_Trq_CR_Shaft/1 -> BusCreator1/1  "Trq_CR_Shaft[Nm]"
  BusCreator1/1 -> Out/1  "Shaft_CR"
  Dummy_omega_Delta_CR_Shaft/1 -> BusCreator1/2  "omega_Delta_CR_Shaft[rad|s]"

== system ASM_Traffic_V2X_Complete_Model_2/MDL/Drivetrain/Final_Drive_Assembly/ASMSignalCollector/Shaft_TGCL4WD/Dummy_TGCL4WD_Shaft ==
  BusCreator1 : BusCreator  Inputs=2
  Dummy_Trq_TGCL4WD_Shaft : Constant  Value=0
  Dummy_omega_Delta_TGCL4WD_Shaft : Constant  Value=0
  Out : Outport
  wires:
  BusCreator1/1 -> Out/1  "Shaft_TGCL4WD"
  Dummy_Trq_TGCL4WD_Shaft/1 -> BusCreator1/1  "Trq_TGCL4WD_Shaft[Nm]"
  Dummy_omega_Delta_TGCL4WD_Shaft/1 -> BusCreator1/2  "omega_Delta_TGCL4WD_Shaft[rad|s]"

== system ASM_Traffic_V2X_Complete_Model_2/MDL/Drivetrain/Final_Drive_Assembly/ASMSignalCollector/Transfer_Gearbox/Dummy_Transfer_Gearbox ==
  BusCreator : BusCreator  Inputs=2
  Dummy_Trq_Cage : Constant  Value=0
  Dummy_omega_Shaft : Constant  Value=0
  Out : Outport
  wires:
  Dummy_Trq_Cage/1 -> BusCreator/1  "Trq_In_Transfer_Gearbox[Nm]"
  BusCreator/1 -> Out/1  "TransferGearbox"
  Dummy_omega_Shaft/1 -> BusCreator/2  "omega_Out_Transfer_Gearbox[rad|s]"

== system ASM_Traffic_V2X_Complete_Model_2/MDL/Environment/EnvironmentInterface_In/Drivetrain/Mapping/n_Engine[rpm] ==
  In1 : Inport
  Out1 : Outport
  wires:
  In1/1 -> Out1/1

== system ASM_Traffic_V2X_Complete_Model_2/MDL/Environment/EnvironmentInterface_In/Drivetrain/Mapping/omega_Out_Trm[rad|s] ==
  In1 : Inport
  Out1 : Outport
  wires:
  In1/1 -> Out1/1

== system ASM_Traffic_V2X_Complete_Model_2/MDL/Environment/EnvironmentInterface_In/SoftECU_Engine/Mapping/AEB[0Off|1On]1 ==
  In1 : Inport
  Out1 : Outport
  wires:
  In1/1 -> Out1/1

== system ASM_Traffic_V2X_Complete_Model_2/MDL/Environment/EnvironmentInterface_In/SoftECU_Engine/Mapping/Const_n_Engine_Idle_Set[rpm]1 ==
  In1 : Inport
  Out1 : Outport
  wires:
  In1/1 -> Out1/1

== system ASM_Traffic_V2X_Complete_Model_2/MDL/Environment/EnvironmentInterface_In/SoftECU_Engine/Mapping/FCW[0Off|1On]1 ==
  In1 : Inport
  Out1 : Outport
  wires:
  In1/1 -> Out1/1

== system ASM_Traffic_V2X_Complete_Model_2/MDL/Environment/EnvironmentInterface_In/SoftECU_Engine/Mapping/State_Engine[0|1|2|3|4]_ ==
  In1 : Inport
  Out1 : Outport
  wires:
  In1/1 -> Out1/1

== system ASM_Traffic_V2X_Complete_Model_2/MDL/Environment/EnvironmentInterface_In/Steering/Mapping/Angle_SteeringWheel[deg]1 ==
  In1 : Inport
  Out1 : Outport
  wires:
  In1/1 -> Out1/1

== system ASM_Traffic_V2X_Complete_Model_2/MDL/Environment/EnvironmentInterface_In/Steering/Mapping/Trq_SteeringWheel[Nm]1 ==
  In1 : Inport
  Out1 : Outport
  wires:
  In1/1 -> Out1/1

== system ASM_Traffic_V2X_Complete_Model_2/MDL/Environment/EnvironmentInterface_In/Steering/Mapping/i_Steering_Mean[]1 ==
  In1 : Inport
  Out1 : Outport
  wires:
  In1/1 -> Out1/1

== system ASM_Traffic_V2X_Complete_Model_2/MDL/Environment/EnvironmentInterface_In/Tire/Mapping/Coef_RollingRes_Mean[]1 ==
  In1 : Inport
  Out1 : Outport
  wires:
  In1/1 -> Out1/1

== system ASM_Traffic_V2X_Complete_Model_2/MDL/Environment/EnvironmentInterface_In/Tire/Mapping/CorneringStiffness_Tire_Front[N|rad]1 ==
  In1 : Inport
  Out1 : Outport
  wires:
  In1/1 -> Out1/1

== system ASM_Traffic_V2X_Complete_Model_2/MDL/Environment/EnvironmentInterface_In/Tire/Mapping/CorneringStiffness_Tire_Rear[N|rad]1 ==
  In1 : Inport
  Out1 : Outport
  wires:
  In1/1 -> Out1/1

== system ASM_Traffic_V2X_Complete_Model_2/MDL/Environment/EnvironmentInterface_In/Tire/Mapping/r_Dyn_Tire_Mean[m]1 ==
  In1 : Inport
  Out1 : Outport
  wires:
  In1/1 -> Out1/1

== system ASM_Traffic_V2X_Complete_Model_2/MDL/Environment/EnvironmentInterface_In/VehicleMovement/Mapping/Inertia_z_Vehicle_Total[kgm2]1 ==
  In1 : Inport
  Out1 : Outport
  wires:
  In1/1 -> Out1/1

== system ASM_Traffic_V2X_Complete_Model_2/MDL/Environment/EnvironmentInterface_In/VehicleMovement/Mapping/Pos_x_CoG_Vehicle_Total[m]1 ==
  In1 : Inport
  Out1 : Outport
  wires:
  In1/1 -> Out1/1

== system ASM_Traffic_V2X_Complete_Model_2/MDL/Environment/EnvironmentInterface_In/VehicleMovement/Mapping/m_TotalVehicle[kg]1 ==
  In1 : Inport
  Out1 : Outport
  wires:
  In1/1 -> Out1/1

== system ASM_Traffic_V2X_Complete_Model_2/MDL/Environment/EnvironmentInterface_In/VehicleMovement/Mapping_Acc/a_y_Vehicle_CoG[m|s2]1 ==
  In1 : Inport
  Out1 : Outport
  wires:
  In1/1 -> Out1/1

== system ASM_Traffic_V2X_Complete_Model_2/MDL/Environment/EnvironmentInterface_In/VehicleMovement/Mapping_F/F_x_Aero_CoorSys_V[N]1 ==
  In1 : Inport
  Out1 : Outport
  wires:
  In1/1 -> Out1/1

== system ASM_Traffic_V2X_Complete_Model_2/MDL/Environment/EnvironmentInterface_In/VehicleMovement/Mapping_F/F_x_Vehicle_Gravitational[N]1 ==
  In1 : Inport
  Out1 : Outport
  wires:
  In1/1 -> Out1/1

== system ASM_Traffic_V2X_Complete_Model_2/MDL/Environment/EnvironmentInterface_In/VehicleMovement/Mapping_F/F_z_Vehicle_Gravitational[N]1 ==
  In1 : Inport
  Out1 : Outport
  wires:
  In1/1 -> Out1/1

== system ASM_Traffic_V2X_Complete_Model_2/MDL/Environment/EnvironmentInterface_In/VehicleMovement/Mapping_Pos/RotationMatrix_V_to_E[3x3]1 ==
  In1 : Inport
  Out1 : Outport
  wires:
  In1/1 -> Out1/1

== system ASM_Traffic_V2X_Complete_Model_2/MDL/Environment/EnvironmentInterface_In/VehicleMovement/Mapping_Pos/s_Vehicle[m]1 ==
  In1 : Inport
  Out1 : Outport
  wires:
  In1/1 -> Out1/1

== system ASM_Traffic_V2X_Complete_Model_2/MDL/Environment/EnvironmentInterface_In/VehicleMovement/Mapping_Vel/RollRate_Vehicle_CoG[deg|s]1 ==
  In1 : Inport
  Out1 : Outport
  wires:
  In1/1 -> Out1/1
